simulink model "AAIRVVIRWORK"  (R2020a)
settings: Solver=FixedStepAuto  StartTime=0.0  StopTime=50.0  FixedStep=1e-3  RelTol=1e-3  EnableMultiTasking=on
undefined symbols (not defined in the file): A0, A1, A2, A3, D0, D1, D10, D11, D12, D13, D2, D3, D4, D5, D6, D7, D8, D9, PTA0, PTA1, PTA2, PTB10, PTB11, PTB2, PTB23, PTB3, PTB9, PTC16, PTC17, PTC2, PTC3, PTC4, PTD0, PTD1, PTD2, PTD3
libraries: frdmk64flib x22, etargetslib x11, dspstat3 x1
(part 2 of 2)

== stateflow chart AAIRVVIRWORK/1.1.3 Subroutines/1.1.3.2 PacemakerControl ==
  state AOOR
    state CHARGE
      entry:
      ATR_PACE_CTRL=LOW;
      VENT_PACE_CTRL=LOW;
      PACING_REF_PWM=ATR_DUTY_CYCLE;
      PACE_CHARGE_CTRL=HIGH;
      PACE_GND_CTRL=HIGH;
      Z_ATR_CTRL=LOW;
      Z_VENT_CTRL=LOW;
      ATR_GND_CTRL=HIGH;
      VENT_GND_CTRL=LOW;
      %atrium_output_voltage = atrium_pulse_amplitude;
      %exit:
      %atrium_output_voltage = 0;
    state DISCHARGE
      entry:
      PACE_CHARGE_CTRL=LOW;
      PACE_GND_CTRL=HIGH;
      ATR_PACE_CTRL=HIGH;
      ATR_GND_CTRL=LOW;
      Z_ATR_CTRL=LOW;
      Z_VENT_CTRL=LOW;
      VENT_GND_CTRL=LOW;
      VENT_PACE_CTRL=LOW;
      PACING_REF_PWM=ATR_DUTY_CYCLE;
      %atrium_output_voltage = 0;
      %exit:
      %atrium_output_voltage = atrium_pulse_amplitude;
    (default) -> AOOR.CHARGE
    AOOR.DISCHARGE -> AOOR.CHARGE : [after(atrium_pulse_width,msec)]
    AOOR.CHARGE -> AOOR.DISCHARGE : [after(f_aoorInterval-atrium_pulse_width,msec)]
  state AAI
    state initializations
      entry:
      ATR_CMP_REF_PWM = ATR_SENS;
      %atrium_output_voltage  = 0;
      count=0;
    state Hysterisis_mode_ON
      entry:
      count = count +1;
    state Hysterisis_mode_OFF
      entry:
      count=count+1;
    state Pulse
      entry:
      %atrium_output_voltage = atrium_pulse_amplitude;
      ATR_PACE_CTRL=LOW;
      VENT_PACE_CTRL=LOW;
      PACING_REF_PWM=ATR_DUTY_CYCLE;
      PACE_CHARGE_CTRL=HIGH;
      PACE_GND_CTRL=HIGH;
      Z_ATR_CTRL=LOW;
      Z_VENT_CTRL=LOW;
      ATR_GND_CTRL=HIGH;
      VENT_GND_CTRL=LOW;
    state CHARGE
      entry:
      %atrium_output_voltage = atrium_pulse_amplitude;
      PACE_CHARGE_CTRL=LOW;
      PACE_GND_CTRL=HIGH;
      ATR_PACE_CTRL=HIGH;
      ATR_GND_CTRL=LOW;
      Z_ATR_CTRL=LOW;
      Z_VENT_CTRL=LOW;
      VENT_GND_CTRL=LOW;
      VENT_PACE_CTRL=LOW;
      PACING_REF_PWM=ATR_DUTY_CYCLE;
      %||((count>WaitTime) && (dig_atr_outputD0 == LOW))
    (default) -> AAI.initializations
    AAI.initializations -> AAI.Hysterisis_mode_ON [order 2] : [hysterisis_flag==1 && after(wait_time_LRL, msec)]
    AAI.initializations -> AAI.Hysterisis_mode_OFF [order 1] : [hysterisis_flag==0 && after(wait_time_LRL, msec)]
    AAI.Pulse -> AAI.initializations : [after(a_r_p,msec)]
    AAI.Hysterisis_mode_ON -> AAI.Hysterisis_mode_ON [order 2] : [(count<=WaitTime)&&(~(dig_atr_outputD0 == LOW && inst_heart_rate<lower_rate_limit))]
    AAI.Hysterisis_mode_OFF -> AAI.Hysterisis_mode_OFF [order 1] : [(count<=WaitTime)&&(~(dig_atr_outputD0 == LOW && inst_heart_rate<lower_rate_limit))]
    AAI.Hysterisis_mode_ON -> AAI.CHARGE [order 1] : [(dig_atr_outputD0 == LOW && inst_heart_rate<h_r_l)]
    AAI.Hysterisis_mode_OFF -> AAI.CHARGE [order 2] : [(dig_atr_outputD0 == LOW && inst_heart_rate<lower_rate_limit)]
    AAI.CHARGE -> AAI.Pulse : [after(atrium_pulse_width,msec)]
  state AAIR
    state initializations
      entry:
      ATR_CMP_REF_PWM = ATR_SENS;
      %atrium_output_voltage  = 0;
    state Hysterisis_mode_ON
      entry:
    state Hysterisis_mode_OFF
      entry:
    state Pulse
      entry:
      %atrium_output_voltage = atrium_pulse_amplitude;
      ATR_PACE_CTRL=LOW;
      VENT_PACE_CTRL=LOW;
      PACING_REF_PWM=ATR_DUTY_CYCLE;
      PACE_CHARGE_CTRL=HIGH;
      PACE_GND_CTRL=HIGH;
      Z_ATR_CTRL=LOW;
      Z_VENT_CTRL=LOW;
      ATR_GND_CTRL=HIGH;
      VENT_GND_CTRL=LOW;
    state CHARGE
      entry:
      %atrium_output_voltage = atrium_pulse_amplitude;
      PACE_CHARGE_CTRL=LOW;
      PACE_GND_CTRL=HIGH;
      ATR_PACE_CTRL=HIGH;
      ATR_GND_CTRL=LOW;
      Z_ATR_CTRL=LOW;
      Z_VENT_CTRL=LOW;
      VENT_GND_CTRL=LOW;
      VENT_PACE_CTRL=LOW;
      PACING_REF_PWM=ATR_DUTY_CYCLE;
      %||((count>WaitTime) && (dig_atr_outputD0 == LOW))
    (default) -> AAIR.initializations
    AAIR.initializations -> AAIR.Hysterisis_mode_ON [order 2] : [hysterisis_flag==1 && after(WaitTimeAAIR, msec)]
    AAIR.initializations -> AAIR.Hysterisis_mode_OFF [order 1] : [hysterisis_flag==0 && after(WaitTimeAAIR, msec)]
    AAIR.Pulse -> AAIR.initializations : [after(a_r_p,msec)]
    AAIR.Hysterisis_mode_ON -> AAIR.CHARGE : [(dig_atr_outputD0 == LOW  && inst_heart_rate<(CurrentRate-5))]
    AAIR.Hysterisis_mode_OFF -> AAIR.CHARGE : [(dig_atr_outputD0 == LOW  && inst_heart_rate<CurrentRate)]
    AAIR.CHARGE -> AAIR.Pulse : [after(atrium_pulse_width,msec)]
  state AOO
    state CHARGE
      entry:
      ATR_PACE_CTRL=LOW;
      VENT_PACE_CTRL=LOW;
      PACING_REF_PWM=ATR_DUTY_CYCLE;
      PACE_CHARGE_CTRL=HIGH;
      PACE_GND_CTRL=HIGH;
      Z_ATR_CTRL=LOW;
      Z_VENT_CTRL=LOW;
      ATR_GND_CTRL=HIGH;
      VENT_GND_CTRL=LOW;
      %atrium_output_voltage = atrium_pulse_amplitude;
      %exit:
      %atrium_output_voltage = 0;
    state DISCHARGE
      entry:
      PACE_CHARGE_CTRL=LOW;
      PACE_GND_CTRL=HIGH;
      ATR_PACE_CTRL=HIGH;
      ATR_GND_CTRL=LOW;
      Z_ATR_CTRL=LOW;
      Z_VENT_CTRL=LOW;
      VENT_GND_CTRL=LOW;
      VENT_PACE_CTRL=LOW;
      PACING_REF_PWM=ATR_DUTY_CYCLE;
      %atrium_output_voltage = 0;
      %exit:
      %atrium_output_voltage = atrium_pulse_amplitude;
    (default) -> AOO.CHARGE
    AOO.DISCHARGE -> AOO.CHARGE : [after(atrium_pulse_width,msec)]
    AOO.CHARGE -> AOO.DISCHARGE : [after(f_aooInterval-atrium_pulse_width,msec)]
  state Initialize
    entry:
    AOO = 100;
    VOO = 200;
    AAI = 112;
    VVI = 222;
    AOOR = 1000;
    AAIR = 1120;
    VOOR = 2000;
    VVIR = 2220;
  state Standby
    entry:
    atrium_output_voltage = 0;
    ventricle_output_voltage = 0;
  state VVI
    state initializations
      entry:
      VENT_CMP_REF_PWM = VENT_SENS;
      %ventricle_output_voltage  = 0;
      count=0;
    state Hysterisis_mode_OFF
      entry:
      count=count+1
    state Pulse
      entry:
      %ventricle_output_voltage = ventricle_pulse_amplitude;
      ATR_PACE_CTRL=LOW;
      VENT_PACE_CTRL=LOW;
      PACING_REF_PWM=VENT_DUTY_CYCLE;
      PACE_CHARGE_CTRL=HIGH;
      PACE_GND_CTRL=HIGH;
      Z_ATR_CTRL=LOW;
      Z_VENT_CTRL=LOW;
      ATR_GND_CTRL=LOW;
      VENT_GND_CTRL=HIGH;
    state Hysterisis_mode_ON
      entry:
      count = count +1;
    state CHARGE
      entry:
      %ventricle_output_voltage = ventricle_pulse_amplitude;
      PACE_CHARGE_CTRL=LOW;
      PACE_GND_CTRL=HIGH;
      ATR_PACE_CTRL=LOW;
      ATR_GND_CTRL=LOW;
      Z_ATR_CTRL=LOW;
      Z_VENT_CTRL=LOW;
      VENT_GND_CTRL=LOW;
      VENT_PACE_CTRL=HIGH;
      PACING_REF_PWM=VENT_DUTY_CYCLE;
      %||((count>WaitTime) && (dig_vent_outputD1 == LOW))
    (default) -> VVI.initializations
    VVI.initializations -> VVI.Hysterisis_mode_ON [order 2] : [hysterisis_flag==1 && after(wait_time_LRL, msec)]
    VVI.initializations -> VVI.Hysterisis_mode_OFF [order 1] : [hysterisis_flag==0 && after(wait_time_LRL, msec)]
    VVI.Pulse -> VVI.initializations : [after(v_r_p,msec)]
    VVI.Hysterisis_mode_OFF -> VVI.Hysterisis_mode_OFF [order 1] : [(count<=WaitTime)&&(~(dig_vent_outputD1 == LOW && inst_heart_rate<lower_rate_limit))]
    VVI.Hysterisis_mode_ON -> VVI.Hysterisis_mode_ON [order 2] : [(count<=WaitTime)&&(~(dig_vent_outputD1 == LOW && inst_heart_rate<lower_rate_limit))]
    VVI.Hysterisis_mode_OFF -> VVI.CHARGE [order 2] : [(dig_vent_outputD1 == LOW && inst_heart_rate<lower_rate_limit)]
    VVI.Hysterisis_mode_ON -> VVI.CHARGE [order 1] : [(dig_vent_outputD1 == LOW && inst_heart_rate<h_r_l)]
    VVI.CHARGE -> VVI.Pulse : [after(ventricle_pulse_width,msec)]
  state VOO
    state CHARGE
      entry:
      ATR_PACE_CTRL=LOW;
      VENT_PACE_CTRL=LOW;
      PACING_REF_PWM=VENT_DUTY_CYCLE;
      PACE_CHARGE_CTRL=HIGH;
      PACE_GND_CTRL=HIGH;
      Z_ATR_CTRL=LOW;
      Z_VENT_CTRL=LOW;
      ATR_GND_CTRL=LOW;
      VENT_GND_CTRL=HIGH;
      %atrium_output_voltage = atrium_pulse_amplitude;
      %exit:
      %atrium_output_voltage = 0;
    state DISCHARGE
      entry:
      PACE_CHARGE_CTRL=LOW;
      PACE_GND_CTRL=HIGH;
      ATR_PACE_CTRL=LOW;
      ATR_GND_CTRL=LOW;
      Z_ATR_CTRL=LOW;
      Z_VENT_CTRL=LOW;
      VENT_GND_CTRL=LOW;
      VENT_PACE_CTRL=HIGH;
      PACING_REF_PWM=VENT_DUTY_CYCLE;
      %ventricle_output_voltage = 0;
      %exit:
      %ventricle_output_voltage = ventricle_pulse_amplitude;
    (default) -> VOO.CHARGE
    VOO.DISCHARGE -> VOO.CHARGE : [after(ventricle_pulse_width,msec)]
    VOO.CHARGE -> VOO.DISCHARGE : [after(f_vooInterval-ventricle_pulse_width,msec)]
  state VVIR
    state initializations
      entry:
      VENT_CMP_REF_PWM = VENT_SENS;
    state Hysterisis_mode_ON
      entry:
    state Hysterisis_mode_OFF
      entry:
    state Pulse
      entry:
      %atrium_output_voltage = atrium_pulse_amplitude;
      ATR_PACE_CTRL=LOW;
      VENT_PACE_CTRL=LOW;
      PACING_REF_PWM=VENT_DUTY_CYCLE;
      PACE_CHARGE_CTRL=HIGH;
      PACE_GND_CTRL=HIGH;
      Z_ATR_CTRL=LOW;
      Z_VENT_CTRL=LOW;
      ATR_GND_CTRL=LOW;
      VENT_GND_CTRL=HIGH;
    state CHARGE
      entry:
      %atrium_output_voltage = atrium_pulse_amplitude;
      PACE_CHARGE_CTRL=LOW;
      PACE_GND_CTRL=HIGH;
      ATR_PACE_CTRL=LOW;
      ATR_GND_CTRL=LOW;
      Z_ATR_CTRL=LOW;
      Z_VENT_CTRL=LOW;
      VENT_GND_CTRL=LOW;
      VENT_PACE_CTRL=HIGH;
      PACING_REF_PWM=VENT_DUTY_CYCLE;
    (default) -> VVIR.initializations
    VVIR.initializations -> VVIR.Hysterisis_mode_ON [order 2] : [hysterisis_flag==1 && after(WaitTimeAAIR, msec)]
    VVIR.initializations -> VVIR.Hysterisis_mode_OFF [order 1] : [hysterisis_flag==0 && after(WaitTimeAAIR, msec)]
    VVIR.Pulse -> VVIR.initializations : [after(v_r_p,msec)]
    VVIR.Hysterisis_mode_ON -> VVIR.CHARGE : [(dig_vent_outputD1 == LOW  && inst_heart_rate<(CurrentRate-5))]
    VVIR.Hysterisis_mode_OFF -> VVIR.CHARGE : [(dig_vent_outputD1 == LOW  && inst_heart_rate<CurrentRate)]
    VVIR.CHARGE -> VVIR.Pulse : [after(ventricle_pulse_width,msec)]
  state VOOR
    state CHARGE
      entry:
      ATR_PACE_CTRL=LOW;
      VENT_PACE_CTRL=LOW;
      PACING_REF_PWM=VENT_DUTY_CYCLE;
      PACE_CHARGE_CTRL=HIGH;
      PACE_GND_CTRL=HIGH;
      Z_ATR_CTRL=LOW;
      Z_VENT_CTRL=LOW;
      ATR_GND_CTRL=LOW;
      VENT_GND_CTRL=HIGH;
      %atrium_output_voltage = atrium_pulse_amplitude;
      %exit:
      %atrium_output_voltage = 0;
    state DISCHARGE
      entry:
      PACE_CHARGE_CTRL=LOW;
      PACE_GND_CTRL=HIGH;
      ATR_PACE_CTRL=LOW;
      ATR_GND_CTRL=LOW;
      Z_ATR_CTRL=LOW;
      Z_VENT_CTRL=LOW;
      VENT_GND_CTRL=LOW;
      VENT_PACE_CTRL=HIGH;
      PACING_REF_PWM=VENT_DUTY_CYCLE;
      %ventricle_output_voltage = 0;
      %exit:
      %ventricle_output_voltage = ventricle_pulse_amplitude;
    (default) -> VOOR.CHARGE
    VOOR.DISCHARGE -> VOOR.CHARGE : [after(ventricle_pulse_width,msec)]
    VOOR.CHARGE -> VOOR.DISCHARGE : [after(f_aoorInterval-ventricle_pulse_width,msec)]
  AOOR -> Standby : [mode ~= AOOR]
  Standby -> AOOR [order 2] : [mode == AOOR]
  AOO -> Standby : [mode ~= AOO]
  Standby -> AOO [order 1] : [mode == AOO]
  AAI -> Standby : [mode ~= AAI]
  Standby -> AAI [order 8] : [mode == AAI]
  AAIR -> Standby : [mode ~= AAIR]
  Standby -> AAIR [order 5] : [mode == AAIR]
  (default) -> Initialize
  Initialize -> Standby : [HR_Ready == true]
  Standby -> Initialize [order 9] : [HR_Ready == false]
  VOO -> Standby : [mode ~= VOO]
  Standby -> VOO [order 7] : [mode == VOO]
  VOOR -> Standby : [mode ~= VOOR]
  Standby -> VOOR [order 4] : [mode == VOOR]
  VVIR -> Standby : [mode ~= VVIR]
  Standby -> VVIR [order 3] : [mode == VVIR]
  VVI -> Standby : [mode ~= VVI]
  Standby -> VVI [order 6] : [mode == VVI]
  data: mode input uint32; upper_rate_limit input uint32; lower_rate_limit input uint32; atrium_pulse_width input double; ventricle_pulse_width input double; f_aooInterval input single; f_vooInterval input single; atrium_output_voltage output single; ventricle_output_voltage output single; AAI local uint32; VVI local uint32; VOO local int32; AOO local uint32; WaitTime input; dig_vent_outputD1 input; avg_heart_rate input; inst_heart_rate input; dig_atr_outputD0 input; hysterisis_flag input; v_r_p input; a_r_p input; prev_inst_heart_rate input; h_r_l input; ATR_GND_CTRL output; ATR_PACE_CTRL output; PACE_CHARGE_CTRL output; PACE_GND_CTRL output; PACING_REF_PWM output; VENT_GND_CTRL output; VENT_PACE_CTRL output; Z_ATR_CTRL output; Z_VENT_CTRL output; HIGH input; LOW input; ATR_DUTY_CYCLE input; VENT_DUTY_CYCLE input; ATR_CMP_REF_PWM output; VENT_CMP_REF_PWM output; VENT_SENS input; ATR_SENS input; HR_Ready input boolean; count output; p_v_a_r_p input; wait_time_hys input; wait_time_LRL input; activity_index input; Recovery_Time input; MSRate input; Reaction_Time input; RF input; f_aoorInterval input; AOOR local; VVIR local; VOOR local; AAIR local; VLOW local; VHIGH local; MHIGH local; MED local; LLOW local; HHIGH local; ActivityThreshold input; XXIR_PPM input; WaitTimeAAIR input; CurrentRate input

== stateflow chart AAIRVVIRWORK/1.1.2 InputProcessing/Activity Index Determination ==
  state init
    entry:
    a = activity_magnitude;
  state V_Low
    entry:
    ActivityIndex = 1
  state Low
    entry:
    ActivityIndex = 2
  state Med_Low
    entry:
    ActivityIndex = 3
  state Med
    entry:
    ActivityIndex = 4
  state Med_High
    entry:
    ActivityIndex = 5
  state High
    entry:
    ActivityIndex = 6
  state V_High
    entry:
    ActivityIndex = 7
  (default) -> init
  init -> V_Low [order 1] : [a >= 0 && a < 1]
  init -> High [order 6] : [a >= 5 && a < 6]
  init -> V_High [order 7] : [a >= 6 && a < 7]
  init -> Low [order 2] : [a >= 1 && a < 2]
  init -> Med_High [order 5] : [a >=4 && a < 5]
  init -> Med_Low [order 3] : [a >= 2 && a < 3]
  init -> Med [order 4] : [a >=3 && a < 4]
  data: activity_magnitude input; ActivityIndex output; a local

== stateflow chart AAIRVVIRWORK/1.1.2 InputProcessing/1.1.2.1 PulsePeriodDetermination ==
  state default
    entry:
  state UnsensedModes
    entry:
    HR_Ready = true
    exit:
    HR_Ready = false
  state AtrialRateDetection1
    state default
      entry:
      pulse_finished = false
      time_between_pulses = 0
    state setARPasDeltaT
      entry:
      time_between_pulses = ARP
    state awaitNewPulse
      entry:
      time_between_pulses = time_between_pulses+1
    state newPulseDetected
      entry:
      pulse_finished = true
      HR_Ready = true
    state resetDeltaT
      entry:
      pulse_finished = false
      time_between_pulses = ARP
    (default) -> AtrialRateDetection1.default
    AtrialRateDetection1.default -> AtrialRateDetection1.setARPasDeltaT : [AtrialPulseDetected == 1]
    AtrialRateDetection1.setARPasDeltaT -> (junction 131) : [after(ARP,msec)]
    AtrialRateDetection1.awaitNewPulse -> AtrialRateDetection1.awaitNewPulse [order 1] : [AtrialPulseDetected == 0]
    (junction 131) -> AtrialRateDetection1.awaitNewPulse [order 1] : [AtrialPulseDetected ==0]
    (junction 131) -> AtrialRateDetection1.newPulseDetected [order 2] : [AtrialPulseDetected == 1]
    AtrialRateDetection1.resetDeltaT -> (junction 131) : [after(ARP-1,msec)]
    AtrialRateDetection1.awaitNewPulse -> AtrialRateDetection1.newPulseDetected [order 2] : [AtrialPulseDetected == 1]
    AtrialRateDetection1.newPulseDetected -> AtrialRateDetection1.resetDeltaT : [after(1,msec)]
  state VenticularRateDetection1
    state default
      entry:
      pulse_finished = false
      time_between_pulses = 0
    state setVRPasDeltaT
      entry:
      time_between_pulses = VRP
    state awaitNewPulse
      entry:
      time_between_pulses = time_between_pulses+1
    state newPulseDetected
      entry:
      pulse_finished = true
      HR_Ready = true
    state resetDeltaT
      entry:
      pulse_finished = false
      time_between_pulses = VRP
    (default) -> VenticularRateDetection1.default
    VenticularRateDetection1.default -> VenticularRateDetection1.setVRPasDeltaT : [VentricularPulseDetected == 1]
    VenticularRateDetection1.setVRPasDeltaT -> (junction 114) : [after(VRP,msec)]
    VenticularRateDetection1.awaitNewPulse -> VenticularRateDetection1.awaitNewPulse [order 1] : [VentricularPulseDetected == 0]
    (junction 114) -> VenticularRateDetection1.awaitNewPulse [order 1] : [VentricularPulseDetected ==0]
    (junction 114) -> VenticularRateDetection1.newPulseDetected [order 2] : [VentricularPulseDetected == 1]
    VenticularRateDetection1.resetDeltaT -> (junction 114) : [after(VRP-1,msec)]
    VenticularRateDetection1.awaitNewPulse -> VenticularRateDetection1.newPulseDetected [order 2] : [VentricularPulseDetected == 1]
    VenticularRateDetection1.newPulseDetected -> VenticularRateDetection1.resetDeltaT : [after(1,msec)]
  state AtrialRateDetection
    state default
      entry:
      pulse_finished = false
      time_between_pulses = 0
    state setARPasDeltaT
      entry:
      time_between_pulses = ARP
    state awaitNewPulse
      entry:
      time_between_pulses = time_between_pulses+1
    state newPulseDetected
      entry:
      pulse_finished = true
      HR_Ready = true
    state resetDeltaT
      entry:
      pulse_finished = false
      time_between_pulses = ARP
    (default) -> AtrialRateDetection.default
    AtrialRateDetection.default -> AtrialRateDetection.setARPasDeltaT : [AtrialPulseDetected == 1]
    AtrialRateDetection.setARPasDeltaT -> (junction 59) : [after(ARP,msec)]
    AtrialRateDetection.awaitNewPulse -> AtrialRateDetection.awaitNewPulse [order 1] : [AtrialPulseDetected == 0]
    (junction 59) -> AtrialRateDetection.awaitNewPulse [order 1] : [AtrialPulseDetected ==0]
    (junction 59) -> AtrialRateDetection.newPulseDetected [order 2] : [AtrialPulseDetected == 1]
    AtrialRateDetection.resetDeltaT -> (junction 59) : [after(ARP-1,msec)]
    AtrialRateDetection.awaitNewPulse -> AtrialRateDetection.newPulseDetected [order 2] : [AtrialPulseDetected == 1]
    AtrialRateDetection.newPulseDetected -> AtrialRateDetection.resetDeltaT : [after(1,msec)]
  state VenticularRateDetection
    state default
      entry:
      pulse_finished = false
      time_between_pulses = 0
    state setVRPasDeltaT
      entry:
      time_between_pulses = VRP
    state awaitNewPulse
      entry:
      time_between_pulses = time_between_pulses+1
    state newPulseDetected
      entry:
      pulse_finished = true
      HR_Ready = true
    state resetDeltaT
      entry:
      pulse_finished = false
      time_between_pulses = VRP
    (default) -> VenticularRateDetection.default
    VenticularRateDetection.default -> VenticularRateDetection.setVRPasDeltaT : [VentricularPulseDetected == 1]
    VenticularRateDetection.setVRPasDeltaT -> (junction 93) : [after(VRP,msec)]
    VenticularRateDetection.awaitNewPulse -> VenticularRateDetection.awaitNewPulse [order 1] : [VentricularPulseDetected == 0]
    (junction 93) -> VenticularRateDetection.awaitNewPulse [order 1] : [VentricularPulseDetected ==0]
    (junction 93) -> VenticularRateDetection.newPulseDetected [order 2] : [VentricularPulseDetected == 1]
    VenticularRateDetection.resetDeltaT -> (junction 93) : [after(VRP-1,msec)]
    VenticularRateDetection.awaitNewPulse -> VenticularRateDetection.newPulseDetected [order 2] : [VentricularPulseDetected == 1]
    VenticularRateDetection.newPulseDetected -> VenticularRateDetection.resetDeltaT : [after(1,msec)]
  (default) -> default
  default -> UnsensedModes [order 4] : [Mode == 100 || Mode == 200]
  VenticularRateDetection1 -> default : [Mode ~= (2220)]
  default -> VenticularRateDetection1 [order 2] : [Mode == 2220]
  AtrialRateDetection1 -> default : [Mode ~= 1120]
  UnsensedModes -> default : [Mode ~= 100 && Mode ~= 200]
  default -> AtrialRateDetection1 [order 3] : [Mode == 1120]
  default -> AtrialRateDetection [order 1] : [Mode == 112]
  AtrialRateDetection -> default : [Mode ~= 112]
  default -> VenticularRateDetection [order 5] : [Mode == 222]
  VenticularRateDetection -> default : [Mode ~= (222)]
  data: Mode input; time_between_pulses output uint32; pulse_finished output boolean; AtrialPulseDetected input boolean; VentricularPulseDetected input boolean; VRP input uint32; ARP input uint32; HR_Ready output boolean

== stateflow chart AAIRVVIRWORK/1.1.1 HardwareInputMapping/HeartChamberPulseDetection ==
  state default
    entry:
    LED_STATE = false
  state led_on
    entry:
    LED_STATE = true
  (default) -> default
  default -> led_on : [in_voltage ==1]
  led_on -> default : [in_voltage ~= 1]
  data: LED_STATE output boolean; in_voltage input

== stateflow chart AAIRVVIRWORK/1.1.1 HardwareInputMapping/HeartChamberPulseDetection3 ==
  state default
    entry:
    LED_STATE = false
  state led_on
    entry:
    LED_STATE = true
  (default) -> default
  default -> led_on : [after(50,msec)]
  led_on -> default : [after(50,msec)]
  data: LED_STATE output boolean

== stateflow chart AAIRVVIRWORK/1.1.1 HardwareInputMapping/HeartChamberPulseDetection2 ==
  state default
    entry:
    LED_STATE = 0
  state led_on
    entry:
    LED_STATE = 1
  (default) -> default
  default -> led_on : [after(10,sec)]
  led_on -> default : [after(10,sec)]
  data: LED_STATE output uint8

== stateflow chart AAIRVVIRWORK/1.1.1 HardwareInputMapping/Chart1 ==
  state Write_Data
    % Set new values for parameters
    entry:
    Mode =Mode_U;
    upper_rate_limit = upper_rate_limit_U;
    lower_rate_limit = lower_rate_limit_U;
    atrial_amplitude = atrial_amplitude_U;
    atrial_pulse_width = atrial_pulse_width_U;
    ventricular_amplitude = ventricular_amplitude_U;
    ventricular_pulse_width = ventricular_pulse_width_U;
    a_r_p = a_r_p_U;
    p_v_a_r_p = p_v_a_r_p_U;
    h_r_l = h_r_l_U;
    r_s_up = r_s_up_U;
    r_s_down = r_s_down_U;
    %ventricular_sensitivity = ventricular_sensitivity_U;
    ventricular_sensitivity = 2.5
    %atrial_sensitivity = atrial_sensitivity_U
    atrial_sensitivity = 2.75
    v_r_p = v_r_p_U;
    hysterisis_flag = hysterisis_flag_U; % should talk about it
    activity_threshold = activity_threshold_U;
    ReactionTime = ReactionTime_U;
    ResponseFactor = ResponseFactor_U;
    RecoveryTime = RecoveryTime_U;
    MSR = MSR_U;
  state setToZeroForTesting
    % Set default values for parameters
    entry:
  state Safety_Check
    entry:
    safety_flag = true;
    while(safety_flag == true)
    if  (~(50<=upper_rate_limit_U<=175))
    safety_flag = false;
    end
    if  (~(50<=lower_rate_limit_U<=upper_rate_limit))
    safety_flag = false;
    end
    if (Mode_U ~= 100 && Mode_U ~= 200 && Mode_U ~= 112 && Mode_U ~= 222 && Mode_U ~= 1000 && Mode_U ~= 1120 && Mode_U ~= 2000 && Mode_U ~= 2220 && Mode_U ~= 3330)
    safety_flag = false;
    end
    if (Mode_U == 100  && lower_rate_limit_U ==60 && atrial_pulse_width_U == 0.4 && a_r_p_U == 250)
    safety_flag = false;
    end
    break
    end
    %Add more input handling errorchecks here
  state Initial_State
    % Set default values for parameters
    entry:
    Mode = 100;
    upper_rate_limit = 175;
    lower_rate_limit = 60;
    atrial_amplitude = 3.75;
    atrial_pulse_width = 0.4;
    ventricular_amplitude = 3.75;
    ventricular_pulse_width = 1;
    a_r_p = 250;
    p_v_a_r_p = 250;
    h_r_l = 45;
    r_s_up = 0.09;
    r_s_down = 0.09;
    ventricular_sensitivity = 2.5;
    atrial_sensitivity = 2.75
    v_r_p = 320;
    hysterisis_flag = 0; % should talk about it
    activity_threshold = 2;
    ReactionTime = 10;
    ResponseFactor = 6;
    RecoveryTime = 2;
    MSR = 120;
  state Read_Data
    entry:
    % --- uint32 (4 bytes) ---
    tmp_u32 = typecast(uint8(rx_data(3:6)), 'uint32'); Mode_U = tmp_u32(1);
    tmp_u32 = typecast(uint8(rx_data(7:10)), 'uint32');   upper_rate_limit_U = tmp_u32(1);
    tmp_u32 = typecast(uint8(rx_data(11:14)), 'uint32');  lower_rate_limit_U = tmp_u32(1);
    tmp_u32 = typecast(uint8(rx_data(39:42)), 'uint32');  a_r_p_U = tmp_u32(1);
    tmp_u32 = typecast(uint8(rx_data(43:46)), 'uint32');  p_v_a_r_p_U = tmp_u32(1);
    tmp_u32 = typecast(uint8(rx_data(47:50)), 'uint32');  h_r_l_U = tmp_u32(1);
    tmp_u32 = typecast(uint8(rx_data(75:78)), 'uint32');  v_r_p_U = tmp_u32(1);
    tmp_u32 = typecast(uint8(rx_data(79:82)), 'uint32');  activity_threshold_U = tmp_u32(1);
    tmp_u32 = typecast(uint8(rx_data(83:86)), 'uint32');  ReactionTime_U = tmp_u32(1);
    tmp_u32 = typecast(uint8(rx_data(87:90)), 'uint32');  ResponseFactor_U = tmp_u32(1);
    tmp_u32 = typecast(uint8(rx_data(91:94)), 'uint32');  RecoveryTime_U = tmp_u32(1);
    tmp_u32 = typecast(uint8(rx_data(95:98)), 'uint32');  MSR_U = tmp_u32(1);
    % --- uint8 (1 byte) ---
    hysterisis_flag_U = uint8(rx_data(99));
    % --- single (float32, 4 bytes) ---
    tmp_single = typecast(uint8(rx_data(15:18)), 'single');  atrial_amplitude_U = tmp_single(1);
    tmp_single = typecast(uint8(rx_data(27:30)), 'single');  ventricular_amplitude_U = tmp_single(1);
    tmp_single = typecast(uint8(rx_data(67:70)), 'single');  atrial_sensitivity_U = tmp_single(1);
    tmp_single = typecast(uint8(rx_data(71:74)), 'single');  ventricular_sensitivity_U = tmp_single(1);
    % --- double (float64, 8 bytes) ---
    tmp_double = typecast(uint8(rx_data(19:26)), 'double');  atrial_pulse_width_U = tmp_double(1);
    tmp_double = typecast(uint8(rx_data(31:38)), 'double');  ventricular_pulse_width_U = tmp_double(1);
    tmp_double = typecast(uint8(rx_data(51:58)), 'double');  r_s_up_U = tmp_double(1);
    tmp_double = typecast(uint8(rx_data(59:66)), 'double');  r_s_down_U = tmp_double(1);
  state Standby
    entry:
    Handshake_Request = 0;
  state HandshakeRequestEnable
    entry:
    Handshake_Request = 1;
  Safety_Check -> Write_Data [order 2] : [safety_flag == true]
  Write_Data -> (junction 81)
  Safety_Check -> setToZeroForTesting [order 1] : [safety_flag == false]
  setToZeroForTesting -> (junction 81)
  (junction 81) -> Standby
  (default) -> Initial_State
  Initial_State -> Standby
  Standby -> (junction 7) : [status==0]
  (junction 12) -> Read_Data [order 1] : [[rx_data(2) == hex2dec('55')]]
  (junction 7) -> (junction 12) : [[rx_data(1) == hex2dec('16')]]
  (junction 12) -> HandshakeRequestEnable [order 2] : [[[rx_data(2) == hex2dec('45')]]]
  HandshakeRequestEnable -> Standby : [after(1,msec)]
  Read_Data -> Safety_Check : [after(1,msec)]
  data: rx_data input; MSR output uint32; ReactionTime output uint32; Mode output uint32; RecoveryTime output uint32; ResponseFactor output uint32; a_r_p output uint32; activity_threshold output uint32; atrial_amplitude output single; atrial_pulse_width output; atrial_sensitivity output single; h_r_l output uint32; hysterisis_flag output uint8; lower_rate_limit output uint32; p_v_a_r_p output uint32; r_s_down output; r_s_up output; upper_rate_limit output uint32; v_r_p output uint32; ventricular_amplitude output single; ventricular_pulse_width output; ventricular_sensitivity output single; MSR_U local uint32; Mode_U local; ReactionTime_U local; RecoveryTime_U local; ResponseFactor_U local; a_r_p_U local; activity_threshold_U local; atrial_amplitude_U local; atrial_pulse_width_U local; atrial_sensitivity_U local; h_r_l_U local; hysterisis_flag_U local; lower_rate_limit_U local; p_v_a_r_p_U local; r_s_down_U local; r_s_up_U local; upper_rate_limit_U local; v_r_p_U local; ventricular_amplitude_U local; ventricular_pulse_width_U local; ventricular_sensitivity_U local; tmp_double local size=8 [1..8]; tmp_u32 local size=8 [1..12]; tmp_single local size=4 [1..4]; status input size=1; safety_flag local boolean; Handshake_Request output uint8

== stateflow chart AAIRVVIRWORK/1.1.2 InputProcessing/Chart ==
  state start
    entry:
    DesiredRate = LowerRateLimit;
    CR = LowerRateLimit;
  state default
    entry:
    flag=0;
    during:
    DesiredRate = LowerRateLimit;
    CR = LowerRateLimit;
    stepup=((MSR-LowerRateLimit)/ReactionTime);
    stepdown=((MSR-LowerRateLimit)/(RecoveryTime*60));
  state stepdown
    entry:
    CR=CR-stepdown;
    flag = 0;
  state overThreshold
    entry:
    flag = 1;
    CR = DesiredRate;
    %DesiredRate = MSR;
    during:
    DesiredRate = LowerRateLimit + (MSR-LowerRateLimit)*(1-2.718^(-1*ResponseFactor*((4*activity_magnitude) - ActivityThreshold)));
  state STEPUP
    entry:
    CR=CR+stepup;
  (default) -> start
  start -> default
  stepdown -> default [order 2] : [CR <= LowerRateLimit]
  default -> overThreshold : [activity_magnitude >= ActivityThreshold]
  stepdown -> stepdown [order 1] : [after(1,sec)]
  overThreshold -> stepdown [order 1] : [activity_magnitude < ActivityThreshold]
  overThreshold -> STEPUP [order 2] : [CR<DesiredRate]
  STEPUP -> overThreshold [order 2] : [CR >= DesiredRate]
  STEPUP -> STEPUP [order 1] : [after(1,sec)]
  data: RecoveryTime input; ReactionTime input; activity_magnitude input single; MSR input single; LowerRateLimit input single; ResponseFactor input single; ActivityThreshold input single; flag output uint32; DesiredRate output single; CR output; stepdown local single; stepup output single
